simulink model "CBF_SafetyFilter"  (R2024b)
settings: Solver=ode45  StartTime=0.0  StopTime=60  RelTol=1e-6  AbsTol=1e-8
libraries: simulink_extras x6
settings Model: Creator=LAPTOPASADI  LastModifiedBy=LAPTOPASADI

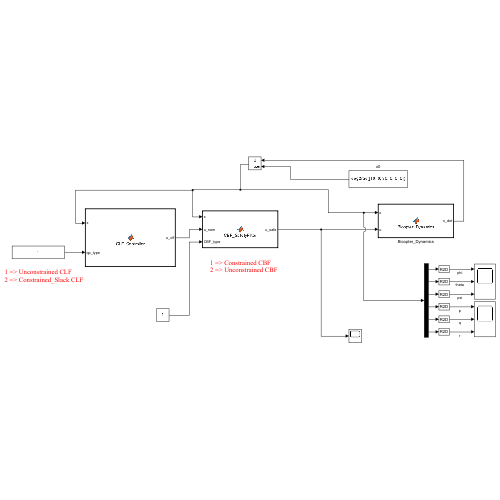
[thumbnail: Simulink's stored preview of the top-level diagram]
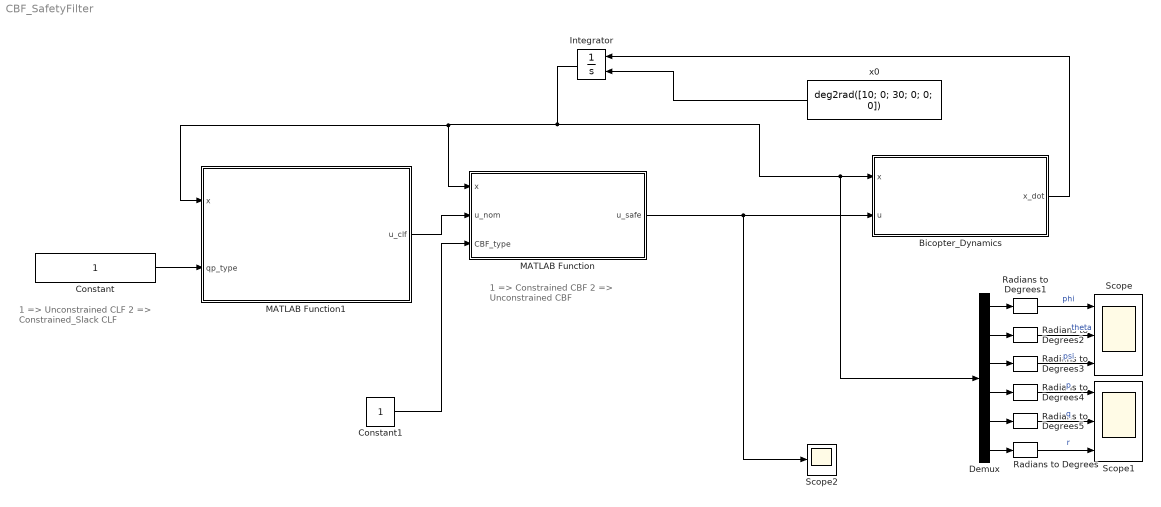
== system CBF_SafetyFilter ==
  note: 1 => Unconstrained CLF
      | 2 => Constrained_Slack CLF
  note: 1 => Constrained CBF
      | 2 => Unconstrained CBF
  Bicopter_Dynamics : MATLAB Function  TreatAsAtomicUnit=on
  Constant : Constant  SampleTime=-1
  Constant1 : Constant
  Demux : Demux  Outputs=6
  Integrator : Integrator  InitialConditionSource=external
  MATLAB Function : MATLAB Function  TreatAsAtomicUnit=on
  MATLAB Function1 : MATLAB Function  TreatAsAtomicUnit=on
  Radians to Degrees{,1..5} (6 alike) : simulink_extras/Transformations/Radians to Degrees
  Scope : Scope  NumInputPorts=3
  Scope1 : Scope  NumInputPorts=3
  Scope2 : Scope
  x0 : Constant  Value=deg2rad([10; 0; 30; 0; 0; 0])  VectorParams1D=off  OutDataTypeStr=double
  wires:
  Bicopter_Dynamics/1(x_dot) -> Integrator/1
  x0/1 -> Integrator/2
  MATLAB Function/1(u_safe) -> Scope2/1, Bicopter_Dynamics/2(u)
  MATLAB Function1/1(u_clf) -> MATLAB Function/2(u_nom)
  Constant/1 -> MATLAB Function1/2(qp_type)
  Integrator/1 -> MATLAB Function1/1(x), MATLAB Function/1(x), Demux/1, Bicopter_Dynamics/1(x)
  Radians to Degrees/1 -> Scope1/3  "r"
  Radians to Degrees5/1 -> Scope1/2  "q"
  Radians to Degrees4/1 -> Scope1/1  "p"
  Radians to Degrees3/1 -> Scope/3  "psi"
  Radians to Degrees2/1 -> Scope/2  "theta"
  Radians to Degrees1/1 -> Scope/1  "phi"
  Demux/4 -> Radians to Degrees4/1
  Demux/3 -> Radians to Degrees3/1
  Demux/6 -> Radians to Degrees/1
  Demux/5 -> Radians to Degrees5/1
  Demux/2 -> Radians to Degrees2/1
  Demux/1 -> Radians to Degrees1/1
  Constant1/1 -> MATLAB Function/3(CBF_type)

== matlab function CBF_SafetyFilter/MATLAB Function ==
  data: x input; u_safe output; u_nom input; CBF_type input
function u_safe = CBF_SafetyFilter(x, u_nom, CBF_type)
% CBF_SAFETYFILTER
%% --- Parameters ---
Ixx = 0.0043;  Iyy = 0.0142;  Izz = 0.0176;  Ixz = 0.0001;
I   = [Ixx, 0, -Ixz;
       0,   Iyy, 0;
      -Ixz, 0,   Izz];

dcg      = 0.175;
hcg      = 0.085; 
d_over_b = 1.2e-6 / 3.13e-5;

B_alloc = [0,  0,    dcg,      d_over_b;
           0,  hcg,  0,        0;
           0,  0,    d_over_b, -dcg];

theta_max = deg2rad(20);   % pitch safety limit
alpha1    = 5;
alpha2    = 5;
u_min     = -0.1;
u_max     =  0.1;

%% --- Extract States ---
phi   = x(1);
theta = x(2);
p     = x(4);
q     = x(5);
r     = x(6);
omega = [p; q; r];

%% --- HOCBF: h = theta_max - theta (relative degree 2) ---
J2        = [0,  cos(phi),  -sin(phi)];  
theta_dot = J2 * omega;

psi0 = theta_max - theta;                 % h(x)
psi1 = -theta_dot + alpha1 * psi0;       

%% --- Lie derivatives of psi1 ---
gyro     = I \ cross(omega, I * omega);   % I^{-1}(omega x I*omega)
Lf_psi1  = J2 * gyro + alpha1 * theta_dot;   % scalar
Lg_psi1  = -J2 * (I \ B_alloc);              % 1x4

%% --- Safety Filter QP ---
A_cbf = -Lg_psi1;
b_cbf =  Lf_psi1 + alpha2 * psi1;

H = 2 * eye(4);
f = -2 * u_nom;
lb = u_min * ones(4,1);
ub = u_max * ones(4,1);

opts = optimoptions('quadprog', 'Algorithm', 'active-set', 'Display', 'off', 'MaxIterations', 200);
[u_safe, ~, flag] = quadprog(H, f, A_cbf, b_cbf, [], [], lb, ub, u_nom, opts);

if flag <= 0 || isempty(u_safe)
    u_safe = u_nom;   
end

switch CBF_type

    case 1
            H = 2 * eye(4);
            f = -2 * u_nom;
            lb = u_min * ones(4,1);
            ub = u_max * ones(4,1);
            
            opts = optimoptions('quadprog', 'Algorithm', 'active-set', 'Display', 'off', 'MaxIterations', 200);
            [u_safe, ~, flag] = quadprog(H, f, A_cbf, b_cbf, [], [], lb, ub, u_nom, opts);
            
            if flag <= 0 || isempty(u_safe)
                u_safe = u_nom;   
            end

    case 2
            opts = optimoptions('quadprog', 'Algorithm', 'active-set', 'Display', 'off');
            [u_safe, ~, flag] = quadprog(H, f, A_cbf, b_cbf, [], [], [], [], u_nom, opts);
            
            if flag <= 0 || isempty(u_safe)
                u_safe = u_nom;   
            end
end
end

== matlab function CBF_SafetyFilter/Bicopter_Dynamics ==
  data: x input; u input; x_dot output
function x_dot = Bicopter_Dynamics(x, u)
%% --- System Parameters ---
Ixx = 0.0043;  Iyy = 0.0142;  Izz = 0.0176;  Ixz = 0.0001;
I   = [Ixx, 0, -Ixz;
       0,   Iyy, 0;
      -Ixz, 0,   Izz];

dcg      = 0.175;
hcg      = 0.085;
d_over_b = 1.2e-6 / 3.13e-5;

B_alloc = [0,  0,    dcg,      d_over_b;
           0,  hcg,  0,        0;
           0,  0,    d_over_b, -dcg];

%% --- Extract States ---
phi   = x(1);
theta = x(2);
p     = x(4);
q     = x(5);
r     = x(6);

omega = [p; q; r];

%% --- Euler Rate Matrix J(phi, theta) ---
cth = cos(theta);
if abs(cth) < 1e-6
    cth = sign(cth + 1e-6) * 1e-6;
end
J = [1,  sin(phi)*sin(theta)/cth,  cos(phi)*sin(theta)/cth;
     0,  cos(phi),                 -sin(phi);
     0,  sin(phi)/cth,              cos(phi)/cth];

%% --- State Derivative ---
euler_dot = J * omega;                          % phi_dot, theta_dot, psi_dot
tau_gyro  = -cross(omega, I * omega);           % gyroscopic torque
omega_dot = I \ (tau_gyro + B_alloc * u);       % angular acceleration

x_dot = [euler_dot; omega_dot];                
end

== matlab function CBF_SafetyFilter/MATLAB Function1 ==
  data: x input; u_clf output; qp_type input
function u_clf = CLF_Controller(x, qp_type)
% CLF_CONTROLLER
% Input:  x (6x1) = [phi; theta; psi; p; q; r]
% Output: u_clf (4x1)

%% --- Parameters ---
Ixx = 0.0043;  Iyy = 0.0142;  Izz = 0.0176;  Ixz = 0.0001;
I   = [Ixx, 0, -Ixz;
       0,   Iyy, 0;
      -Ixz, 0,   Izz];

dcg      = 0.175;
hcg      = 0.085;
d_over_b = 1.2e-6 / 3.13e-5;

B_alloc = [0,  0,    dcg,      d_over_b;
           0,  hcg,  0,        0;
           0,  0,    d_over_b, -dcg];

gamma   = 0.5;
u_min   = -0.01;
u_max   =  0.01;

%% --- P matrix hardcoded (pre-computed: lyap(Acl', 0.1*eye(6))) ---
P = [0.11250,       0,       0,   0.01250,       0,       0;
          0,  0.11250,       0,         0,  0.01250,       0;
          0,       0,  0.11250,         0,       0,  0.01250;
     0.01250,      0,       0,   0.01563,       0,       0;
          0,  0.01250,      0,         0,  0.01563,       0;
          0,       0,  0.01250,         0,       0,  0.01563];

%% --- Extract States ---
phi   = x(1);  theta = x(2);  psi = x(3);
p     = x(4);  q     = x(5);  r   = x(6);
omega = [p; q; r];

y     = [phi; theta - deg2rad(30); psi];


%% --- Euler Rate Matrix & augmented state ---
J     = local_J(phi, theta);
y_dot = J * omega;
eta   = [y; y_dot];   % 6x1

%% --- CLF value ---
V = eta' * P * eta;
if V < 1e-8
    u_clf = zeros(4,1);
    return;
end

%% --- Lie Derivatives of V ---
Jdot        = local_Jdot(phi, theta, omega);
tau_gyro    = -cross(omega, I * omega);
omega_drift = I \ tau_gyro;

alpha_vec = Jdot * omega + J * omega_drift;  % 3x1
A_mat     = J * (I \ B_alloc);              % 3x4

f_eta   = [y_dot;      alpha_vec];
g_eta   = [zeros(3,4); A_mat   ];

dV_deta = 2 * eta' * P;
LfV     = dV_deta * f_eta;   % scalar
LgV     = dV_deta * g_eta;   % 1x4

%% --- Slack CLF-QP  (z = [u; delta], 5x1) ---

opts = optimoptions('quadprog','Algorithm','active-set','Display','off','MaxIterations',200);


    switch qp_type
        case 1
            % Original QP without limits
            H = 2 * eye(4);
            fqp = zeros(4,1);
            Aineq = LgV;                  
            bineq = -LfV - gamma * V;      
                z = quadprog(H, fqp, Aineq, bineq, [], [], [], [], zeros(4,1), opts);


        case 2
            
            w_slack = 1e6; 
            
           H     = 2 * diag([1, 1, 1, 1, w_slack]);
           fqp   = zeros(5,1);
           Aineq = [LgV, -1];
           bineq = -LfV - gamma * V;
           lb    = [u_min*ones(4,1); 0  ];
           ub    = [u_max*ones(4,1); Inf];
                        
            z = quadprog(H, fqp, Aineq, bineq, [], [], lb, ub, zeros(5,1), opts);
            
           
        otherwise
            error('Unknown qp_type. Choose unconstrained, constrained_hard, or constrained_slack.');
    end

    if isempty(z)
        u_clf = zeros(4,1);
    else
        u_clf = z(1:4);
    end

end


%%  Local helpers 
function J = local_J(phi, theta)
    cth = cos(theta);
    if abs(cth) < 1e-6,  cth = sign(cth+1e-6)*1e-6;  end
    J = [1,  sin(phi)*sin(theta)/cth,  cos(phi)*sin(theta)/cth;
         0,  cos(phi),                 -sin(phi);
         0,  sin(phi)/cth,              cos(phi)/cth];
end

function Jd = local_Jdot(phi, theta, omega)
    J  = local_J(phi, theta);
    ed = J * omega;
    pd = ed(1);  td = ed(2);
    cth = cos(theta);  sth = sin(theta);
    if abs(cth) < 1e-6,  cth = sign(cth+1e-6)*1e-6;  end
    tth = sth/cth;  sc = 1/cth;  s2 = sc^2;
    dJdphi   = [0,  cos(phi)*tth,       -sin(phi)*tth;
                0, -sin(phi),            -cos(phi);
                0,  cos(phi)*sc,         -sin(phi)*sc];
    dJdtheta = [0,  sin(phi)*s2,          cos(phi)*s2;
                0,  0,                    0;
                0,  sin(phi)*sc*tth,      cos(phi)*sc*tth];
    Jd = dJdphi*pd + dJdtheta*td;
end
